simulink subsystem "bus2vector"  (R2019b)
settings: Solver=VariableStepAuto  StartTime=0.0  StopTime=10.0  RelTol=1e-3
settings Model: Creator=acook  LastModifiedBy=acook

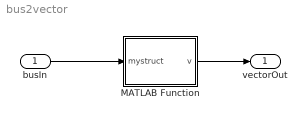
== system bus2vector ==
  busIn : Inport
  MATLAB Function : MATLAB Function  TreatAsAtomicUnit=on
  vectorOut : Outport
  wires:
  busIn/1 -> MATLAB Function/1(mystruct)
  MATLAB Function/1(v) -> vectorOut/1

== matlab function bus2vector/MATLAB Function ==
  data: mystruct input; v output
function v = fcn(mystruct)
%% Assumes each bus element is a vector of the same length


fns = fieldnames(mystruct);

v = zeros(numel(fns),length(mystruct.(fns{1})));

for fn = fns'
    v(k,:) = fn.(fn{:});
end
